simulink model "PI_Sim"  (R2020a)
settings: Solver=FixedStepAuto  StartTime=0.0  StopTime=800  FixedStep=0.1  RelTol=1e-3
undefined symbols (not defined in the file): Td, Ti, Zr
libraries: simulink x1
settings Model: Creator=MK  LastModifiedBy=olive

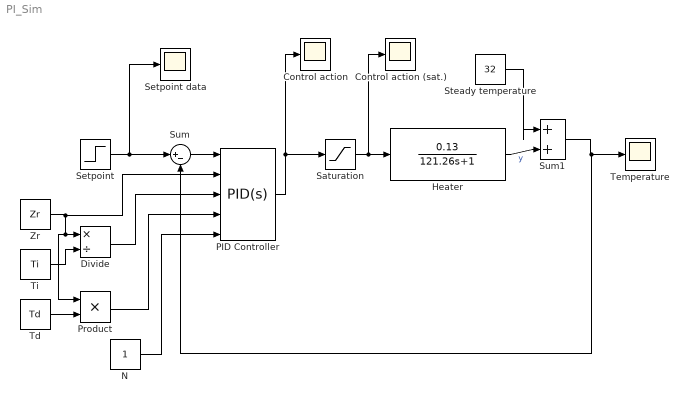
== system PI_Sim ==
  Control action : Scope
  Control action (sat.) : Scope
  Divide : Product  Inputs=*/
  Heater : TransferFcn  Numerator=0.13  Denominator=[121.26 1]
  N : Constant
  PID Controller : simulink/Continuous/PID Controller  Controller=PID  Form=Parallel  TimeDomain=Continuous-time  UseExternalTs=off  SampleTime=-1  IntegratorMethod=Forward Euler  FilterMethod=Forward Euler  ControllerParametersSource=external  P=Zr  I=Zr/Ti  D=Zr*Td  UseFilter=on  N=100  TunerSelectOption=Transfer Function Based (PID Tuner App)  InitialConditionSource=internal  InitialConditionForIntegrator=0  InitialConditionForFilter=0  DifferentiatorICPrevScaledInput=0  ExternalReset=none  TrackingMode=off  Kt=1  LimitOutput=off  UpperSaturationLimit=50  LowerSaturationLimit=-50  LinearizeAsGain=on  AntiWindupMode=clamping  Kb=1  POutMin=[]  POutMax=[]  IOutMin=[]  IOutMax=[]  DOutMin=[]  DOutMax=[]  NOutMin=[]  NOutMax=[]  SumOutMin=[]  SumOutMax=[]  SaturationOutMin=[]  SaturationOutMax=[]  PParamMin=[]  PParamMax=[]  IParamMin=[]  IParamMax=[]  DParamMin=[]  DParamMax=[]  NParamMin=[]  NParamMax=[]  KbParamMin=[]  KbParamMax=[]  KtParamMin=[]  KtParamMax=[]  KbOutMin=[]  KbOutMax=[]  KtOutMin=[]  KtOutMax=[]  IntegratorOutMin=[]  IntegratorOutMax=[]  FilterOutMin=[]  FilterOutMax=[]  SumI1OutMin=[]  SumI1OutMax=[]  SumI2OutMin=[]  SumI2OutMax=[]  SumI3OutMin=[]  SumI3OutMax=[]  SumI4OutMin=[]  SumI4OutMax=[]  SumDOutMin=[]  SumDOutMax=[]  DifferentiatorOutMin=[]  DifferentiatorOutMax=[]  FilterDiffOutCoefMin=[]  FilterDiffOutCoefMax=[]  ReciprocalOutMin=[]  ReciprocalOutMax=[]  SumDenOutMin=[]  SumDenOutMax=[]  SumNumOutMin=[]  SumNumOutMax=[]  DivideOutMin=[]  DivideOutMax=[]  UdiffTsProdOutMin=[]  UdiffTsProdOutMax=[]  NTsProdOutMin=[]  NTsProdOutMax=[]  UintegralTsProdOutMin=[]  UintegralTsProdOutMax=[]  UngainTsProdOutMin=[]  UngainTsProdOutMax=[]  IntegratorContinuousStateAttributes=''  IntegratorStateMustResolveToSignalObject=off  IntegratorRTWStateStorageClass=Auto  FilterContinuousStateAttributes=''  FilterStateMustResolveToSignalObject=off  FilterRTWStateStorageClass=Auto  ParallelPVariant=ExternalParameters  IdealPVariant=Disabled  IVariant=ExternalParameters  DVariant=ExternalParameters  IntegratorVariant=Continuous  SatVariant=Disabled  AWVariant=Passthrough  PCopyVariant=Disabled  TRVariant=Disabled  FdbkBlocksVariant=Forward  IdealPFdbkVariant=Disabled  SatFdbkVariant=Disabled  DerivativeFilterVariant=ContFilter  NVariant=ExternalParameters  NCopyVariant=Disabled  FilterICVariant=InternalICsFilter  IntegratorICVariant=InternalICs  ExternalResetVariant=Disabled  TRSumVariant=Passthrough  SumFdbkVariant=Disabled  SumVariant=Sum_PID  TsampFilterVariant=InternalTs  TsampNgainVariant=Passthrough  TsampIntegralVariant=Passthrough
  Product : Product
  "Saturation " : Saturate  UpperLimit=50  LowerLimit=-50
  Setpoint : Step  Time=10  Before=32  After=35  SampleTime=0
  Setpoint data : Scope
  Steady temperature : Constant  Value=32
  Sum : Sum  Inputs=|+-
  Sum1 : Sum  Inputs=|++
  Td : Constant  Value=Td
  Temperature : Scope
  Ti : Constant  Value=Ti
  Zr : Constant  Value=Zr
  wires:
  Setpoint/1 -> Setpoint data/1, Sum/1
  Sum/1 -> PID Controller/1
  Steady temperature/1 -> Sum1/1
  Heater/1 -> Sum1/2  "y"
  Sum1/1 -> Sum/2, Temperature/1
  N/1 -> PID Controller/5
  Zr/1 -> PID Controller/2, Product/1, Divide/1
  Td/1 -> Product/2
  Ti/1 -> Divide/2
  Divide/1 -> PID Controller/3
  Product/1 -> PID Controller/4
  PID Controller/1 -> "Saturation "/1, Control action/1
  "Saturation "/1 -> Control action (sat.)/1, Heater/1
